simulink model "mic_decimator"  (R2024b)
settings: Solver=FixedStepDiscrete  StartTime=0.0  StopTime=10.0  FixedStep=Tpdm  RelTol=1e-3
PreLoadFcn:
  | if ~exist('Tpdm','var'), iir_setup; end
values from neighbouring files (symbols this model uses):
  Rdec = 64    [iir_setup.m]
  Tpdm = 32/100e6    (= 3.2e-07)    [iir_setup.m]
undefined symbols (not defined in the file or in its folder): DiscIntNeverNeededParam
libraries: dspmlti4 x1
settings Model: Creator=samue  LastModifiedBy=samue
settings DebuggingCC: SingleTaskRateTransMsg=error  IntegerOverflowMsg=none  ParameterPrecisionLossMsg=none

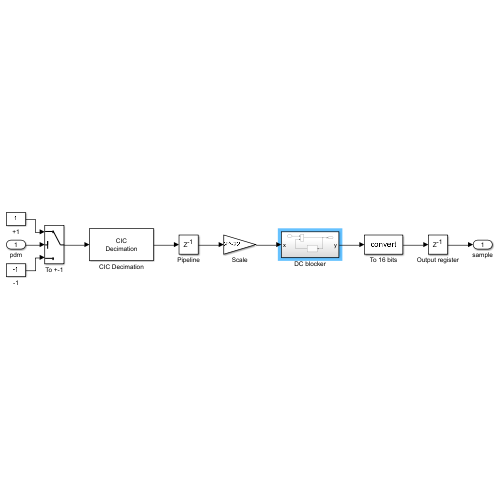
[thumbnail: Simulink's stored preview of the top-level diagram]
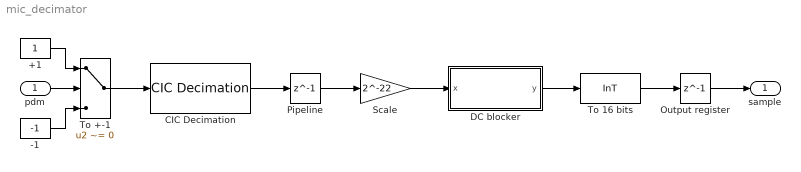
== system mic_decimator ==
  pdm : Inport  OutDataTypeStr=boolean  SampleTime=Tpdm
  +1 : Constant  OutDataTypeStr=fixdt(1,2,0)
  -1 : Constant  Value=-1  OutDataTypeStr=fixdt(1,2,0)
  CIC Decimation : dspmlti4/CIC Decimation  filtFrom=Dialog parameters  filtobj=CICDECIM  ftype=Decimator  R=Rdec  M=1  N=4  filterInternals=Full precision  BPS=[16 16 16 16]  FLPS=0  outputWordLength=32  outputFracLength=0  launchFVT=off  framing=Maintain input frame rate  RateOptions=Allow multirate processing
      settings: LibrarySourceBlock=|
      | dsphdlsupportfiltering/CIC
      | Decimation
  DC blocker : Subsystem
  Output register : Delay  DelayLength=1
  Pipeline : Delay  DelayLength=1
  Scale : Gain  Gain=2^-22  ParamDataTypeStr=fixdt(0,1,22)  OutDataTypeStr=fixdt(1,26,22)
  To +-1 : Switch  Criteria=u2 ~= 0  SaturateOnIntegerOverflow=off  InputSameDT=off
  To 16 bits : DataTypeConversion  OutDataTypeStr=InT  RndMeth=Floor
  sample : Outport
  wires:
  +1/1 -> To +-1/1
  pdm/1 -> To +-1/2
  -1/1 -> To +-1/3
  To +-1/1 -> CIC Decimation/1
  CIC Decimation/1 -> Pipeline/1
  Pipeline/1 -> Scale/1
  Scale/1 -> DC blocker/1(x)
  DC blocker/1(y) -> To 16 bits/1
  To 16 bits/1 -> Output register/1
  Output register/1 -> sample/1

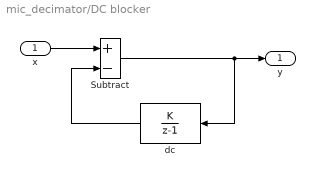
== system mic_decimator/DC blocker ==
  x : Inport
  Subtract : Sum  Inputs=+-  OutDataTypeStr=fixdt(1,27,22)
  dc : DiscreteIntegrator  IntegratorMethod=Accumulation: Forward Euler  gainval=2^-10  SampleTime=-1  OutDataTypeStr=fixdt(1,37,32)  ICPrevOutput=DiscIntNeverNeededParam  ICPrevScaledInput=DiscIntNeverNeededParam
  y : Outport
  wires:
  x/1 -> Subtract/1
  Subtract/1 -> y/1, dc/1
  dc/1 -> Subtract/2
